simulink model "SP_yaw_pid"  (R2013b)
settings: Solver=ode3  StartTime=0.0  StopTime=5  FixedStep=0.001  RelTol=1e-3
settings Model: Creator=Zhaolei  LastModifiedBy=zhaol

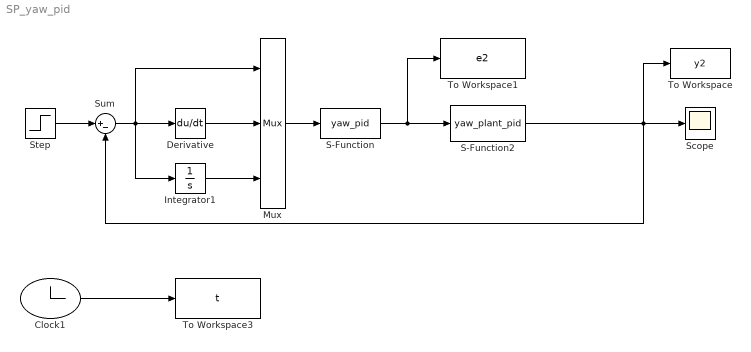
== system SP_yaw_pid ==
  Clock1 : Clock
  Derivative : Derivative
  Integrator1 : Integrator
  Mux : Mux  Inputs=3
  S-Function : S-Function  FunctionName=yaw_pid  EnableBusSupport=off
  S-Function2 : S-Function  FunctionName=yaw_plant_pid  EnableBusSupport=off
  Scope : Scope
  Step : Step  After=0  SampleTime=0
  Sum : Sum  Inputs=|+-
  To Workspace : ToWorkspace  VariableName=y2  SampleTime=-1
  To Workspace1 : ToWorkspace  VariableName=e2  SampleTime=-1
  To Workspace3 : ToWorkspace  VariableName=t  SampleTime=-1
  wires:
  Clock1/1 -> To Workspace3/1
  Step/1 -> Sum/1
  Sum/1 -> Mux/1, Integrator1/1, Derivative/1
  Derivative/1 -> Mux/2
  Integrator1/1 -> Mux/3
  Mux/1 -> S-Function/1
  S-Function/1 -> To Workspace1/1, S-Function2/1
  S-Function2/1 -> To Workspace/1, Sum/2, Scope/1
